simulink model "pwaSys_obs_model_d"  (Simulink 8.6)
settings: Solver=ode45  StartTime=0.0  StopTime=sim_T  RelTol=1e-3
InitFcn:
  | load simulink.mat
  | setParameters
StartFcn:
  | load simulink.mat
  | setParameters
  | clear res_X res_U res_Y res_P res_D
  | clear res_Xest res_Dest res_Yest
StopFcn:
  | plotScope
undefined symbols (not defined in the file or in its folder): sigbuilder_block, sim_d, sim_nd, sim_nx, sim_ny, sim_x0
undefined symbols (not defined in the file): sim_A, sim_Aobs, sim_B, sim_Bobs, sim_C, sim_Cobs, sim_D, sim_d0obs, sim_Dobs, sim_H, sim_Hobs, sim_K, sim_Kobs, sim_Ts, sim_TsObs, sim_x0obs
settings Model: Creator=alberto  LastModifiedBy=root
settings DataIOCC: SignalLoggingSaveFormat=Dataset
settings OptimizationCC: ExpressionDepthLimit=128
settings DebuggingCC: UnderspecifiedInitializationDetection=Simplified  MergeDetectMultiDrivingBlocksExec=error  FcnCallInpInsideContextMsg=EnableAllAsError  StateNameClashWarn=none
settings GRTTargetCC: CombineOutputUpdateFcns=on  GRTInterface=off
settings ConfigComp: CovSFcnEnable=off

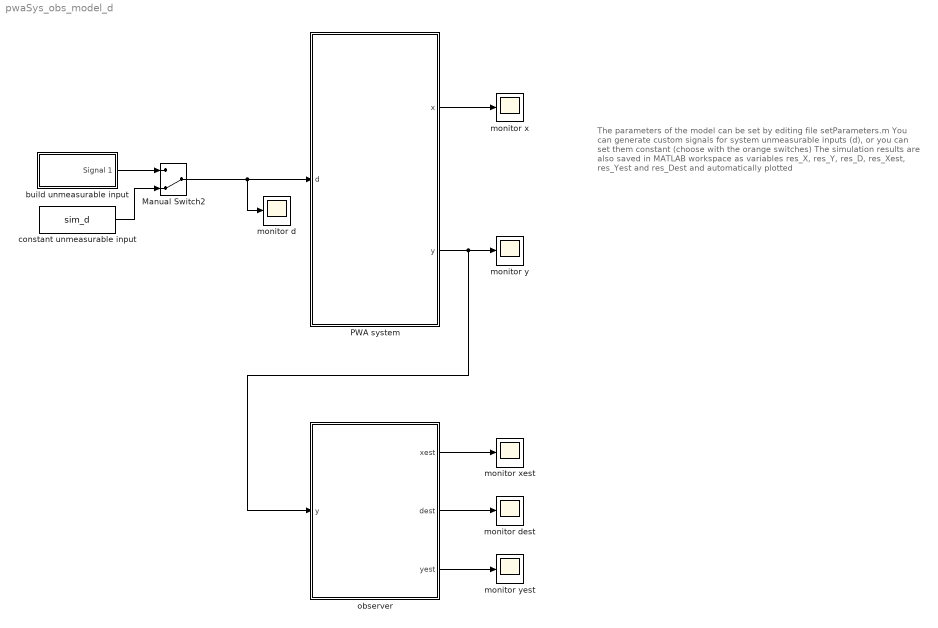
== system pwaSys_obs_model_d ==
  note: The parameters of the model can be set by editing file setParameters.m
      |
      | You can generate custom signals for system unmeasurable inputs (d),
      | or you can set them constant (choose with the orange switches)
      |
      | The simulation results are also saved in MATLAB workspace as variables
      | res_X, res_Y, res_D, res_Xest, res_Yest and res_Dest and
      | automatically plotted
  Manual Switch2 : ManualSwitch  CurrentSetting=0
  PWA system : Subsystem
  build unmeasurable input : Subsystem  Tag=STV Subsys  LoadFcn=sigbuilder_block('load');  StartFcn=sigbuilder_block('start');  StopFcn=sigbuilder_block('stop');  ClipboardFcn=sigbuilder_block('clipboard');  mask(Sigbuilder block){}
      mask help: Simulink:masks:SigbuilderBlock_MD
      mask init:
      | if ~strcmp(get_param(bdroot(gcbh),'SimulationStatus'),'stopped') tuvar = sigbuilder_block('maskInit'); end
      settings: CopyFcn=sigbuilder_block('copy');  DeleteFcn=sigbuilder_block('delete');  ModelCloseFcn=sigbuilder_block('modelClose');  PreSaveFcn=sigbuilder_block('preSave');  PauseFcn=sigbuilder_block('pause');  ContinueFcn=sigbuilder_block('continue');  NameChangeFcn=sigbuilder_block('namechange');  OpenFcn=sigbuilder_block('open',[433.6 121.6 550.4 399.2 ]);  CloseFcn=sigbuilder_block('close');
      mask Display: plot(0, 0, 100, 100,[2, 2, 32, 32, 2], [68, 8, 8, 68, 68],[32, 2], [38, 38], [32, 19, 2],[53, 60, 44], [32, 17, 17, 2],[16, 16, 31, 31]);txt = getActiveGroup(gcbh);text(2, 100, txt,'verticalAlignment', 'top');
  constant unmeasurable input : Constant  Value=sim_d
  monitor d : Scope
  monitor dest : Scope
  monitor x : Scope
  monitor xest : Scope
  monitor y : Scope
  monitor yest : Scope
  observer : Subsystem
  wires:
  PWA system/1(x) -> monitor x/1
  PWA system/2(y) -> observer/1(y), monitor y/1
  build unmeasurable input/1(Signal 1) -> Manual Switch2/1
  constant unmeasurable input/1 -> Manual Switch2/2
  Manual Switch2/1 -> monitor d/1, PWA system/1(d)
  observer/1(xest) -> monitor xest/1
  observer/2(dest) -> monitor dest/1
  observer/3(yest) -> monitor yest/1

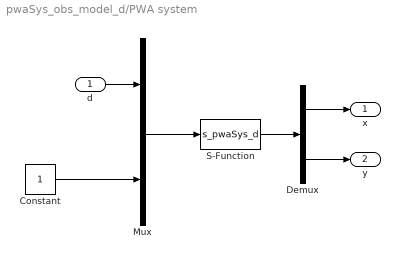
== system pwaSys_obs_model_d/PWA system ==
  d : Inport
  Constant : Constant
  Demux : Demux  Outputs=[sim_nx sim_ny]
  Mux : Mux  Inputs=2
  S-Function : S-Function  FunctionName=s_pwaSys_d  Parameters=A,B,C,D,H,K,sim_x0,Ts  SFunctionDeploymentMode=off  EnableBusSupport=off  mask{A=sim_A, B=sim_B, C=sim_C, D=sim_D, H=sim_H, K=sim_K, sim_x0=sim_x0, Ts=sim_Ts}
      mask prompts: sim_x0 "Initial condition"; Ts "Sample time"
      mask DialogControl DescTextVar Prompt: continuous time PWA system
  x : Outport
  y : Outport  Port=2
  wires:
  d/1 -> Mux/1
  Mux/1 -> S-Function/1
  S-Function/1 -> Demux/1
  Demux/1 -> x/1
  Demux/2 -> y/1
  Constant/1 -> Mux/2

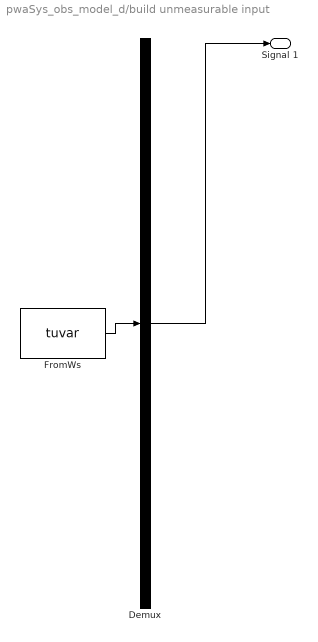
== system pwaSys_obs_model_d/build unmeasurable input ==
  Demux : Demux  Tag=STV Demux  Outputs=1
  FromWs : FromWorkspace  Tag=STV FromWs  VariableName=tuvar  SampleTime=0  SigBuilderData=DataTag0  VnvData=DataTag1
      SigBuilderData=|
      | common.afterFinalStr = 'Extrapolate'
      | common.sampleTime = 0
      | dataSet.timeRange = [0 10]
      | dataSet.name = 'Group 1'
      | sbobj.Groups.Name = 'Group 1'
      | sbobj.Groups.Signals.Name = 'Signal 1'
      | sbobj.Groups.Signals.XData = [0 6 10]
      | sbobj.Groups.Signals.YData = [0 0 0]
  Signal 1 : Outport  Tag=STV Outport
  wires:
  Demux/1 -> Signal 1/1
  FromWs/1 -> Demux/1

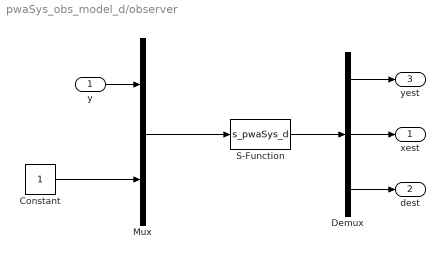
== system pwaSys_obs_model_d/observer ==
  y : Inport
  Constant : Constant
  Demux : Demux  Outputs=[sim_ny sim_nx sim_nd]
  Mux : Mux  Inputs=2
  S-Function : S-Function  FunctionName=s_pwaSys_d  Parameters=A,B,C,D,H,K,sim_x0,Ts  SFunctionDeploymentMode=off  EnableBusSupport=off  mask{A=sim_Aobs, B=sim_Bobs, C=sim_Cobs, D=sim_Dobs, H=sim_Hobs, K=sim_Kobs, sim_x0=[sim_x0obs;sim_d0obs], Ts=sim_TsObs}
      mask prompts: sim_x0 "Initial condition"; Ts "Sample time"
      mask DialogControl DescTextVar Prompt: continuous time PWA system
  xest : Outport
  dest : Outport  Port=2
  yest : Outport  Port=3
  wires:
  Mux/1 -> S-Function/1
  S-Function/1 -> Demux/1
  Constant/1 -> Mux/2
  y/1 -> Mux/1
  Demux/1 -> yest/1
  Demux/2 -> xest/1
  Demux/3 -> dest/1
